simulink model "obstaculo_senoidal"  (R2025a)
settings: Solver=ode45  StartTime=0.0  StopTime=18  RelTol=1e-3
values from neighbouring files (symbols this model uses):
  a2 = entre_eixos - a_Ax    (= 0.114356)    [parametros_suspensao_completo_pibit_final.m]
  a_Ax = 0.070    (= 0.07)    [parametros_suspensao_completo_pibit_final.m]
  Hmax = 10/100    (= 0.1)    [parametros_suspensao_completo_pibit_final.m]
  Lqm = 3,7    [parametros_suspensao_completo_pibit_final.m]
  n_obs = 10    [parametros_suspensao_completo_pibit_final.m]
  Vv = 5    [parametros_suspensao_completo_pibit_final.m]
  Xobs = 10    [parametros_suspensao_completo_pibit_final.m]
libraries: simulink x4

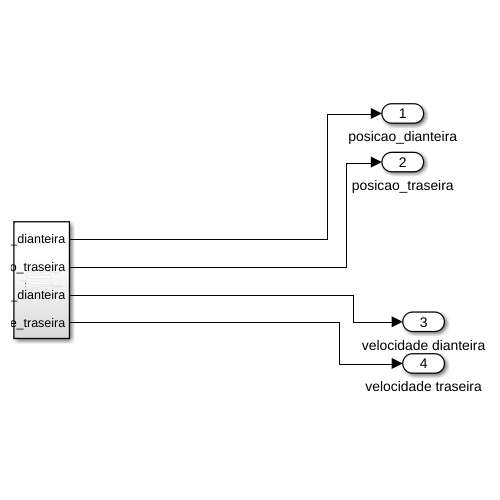
[thumbnail: Simulink's stored preview of the top-level diagram]
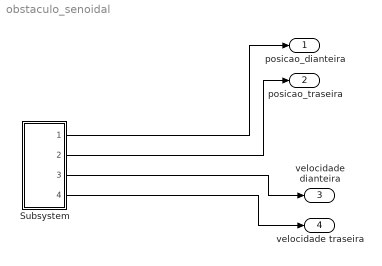
== system obstaculo_senoidal ==
  Subsystem : Subsystem
  posicao_dianteira : Outport
  posicao_traseira : Outport  Port=2
  velocidade dianteira : Outport  Port=3
  velocidade traseira : Outport  Port=4
  wires:
  Subsystem/1(posicao_dianteira) -> posicao_dianteira/1
  Subsystem/2(posicao_traseira) -> posicao_traseira/1
  Subsystem/3(velocidade_dianteira) -> velocidade dianteira/1
  Subsystem/4(velocidade_traseira) -> velocidade traseira/1

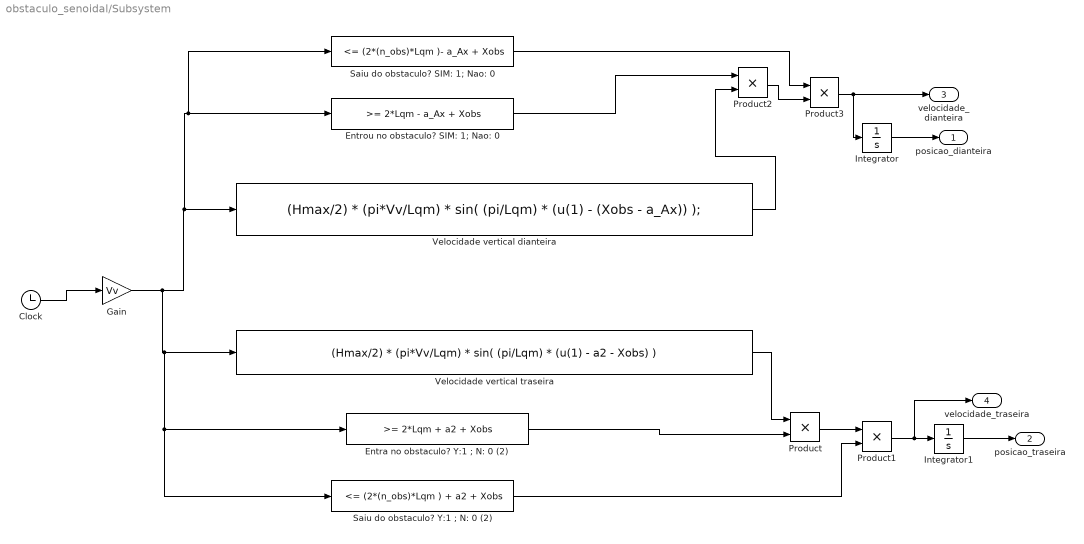
== system obstaculo_senoidal/Subsystem ==
  Clock : Clock
  Entra no obstaculo? Y:1 ; N: 0 (2) : simulink/Logic and Bit Operations/Compare To Constant  relop=>=  const=2*Lqm + a2 + Xobs  OutDataTypeStr=boolean
  "Entrou no obstaculo? SIM: 1; Nao: 0 " : simulink/Logic and Bit Operations/Compare To Constant  relop=>=  const=2*Lqm - a_Ax + Xobs  OutDataTypeStr=boolean
  Gain : Gain  Gain=Vv
  Integrator : Integrator
  Integrator1 : Integrator
  Product{,1..3} (4 alike) : Product
  "Saiu do obstaculo? SIM: 1; Nao: 0 " : simulink/Logic and Bit Operations/Compare To Constant  relop=<=  const=(2*(n_obs)*Lqm )- a_Ax + Xobs  OutDataTypeStr=boolean
  Saiu do obstaculo? Y:1 ; N: 0 (2) : simulink/Logic and Bit Operations/Compare To Constant  relop=<=  const=(2*(n_obs)*Lqm ) + a2 + Xobs  OutDataTypeStr=boolean
  Velocidade vertical dianteira : Fcn  Expr=(Hmax/2) * (pi*Vv/Lqm) * sin( (pi/Lqm) * (u(1) - (Xobs - a_Ax)) );
  Velocidade vertical traseira : Fcn  Expr=(Hmax/2) * (pi*Vv/Lqm) * sin( (pi/Lqm) * (u(1) - a2 - Xobs) )
  posicao_dianteira : Outport
  posicao_traseira : Outport  Port=2
  velocidade_dianteira : Outport  Port=3
  velocidade_traseira : Outport  Port=4
  wires:
  Gain/1 -> Saiu do obstaculo? Y:1 ; N: 0 (2)/1, Entra no obstaculo? Y:1 ; N: 0 (2)/1, Velocidade vertical traseira/1, "Saiu do obstaculo? SIM: 1; Nao: 0 "/1, "Entrou no obstaculo? SIM: 1; Nao: 0 "/1, Velocidade vertical dianteira/1
  Entra no obstaculo? Y:1 ; N: 0 (2)/1 -> Product/2
  "Saiu do obstaculo? SIM: 1; Nao: 0 "/1 -> Product3/1
  Saiu do obstaculo? Y:1 ; N: 0 (2)/1 -> Product1/2
  Product2/1 -> Product3/2
  Product3/1 -> velocidade_dianteira/1, Integrator/1
  Integrator/1 -> posicao_dianteira/1
  Product/1 -> Product1/1
  Velocidade vertical traseira/1 -> Product/1
  Product1/1 -> velocidade_traseira/1, Integrator1/1
  "Entrou no obstaculo? SIM: 1; Nao: 0 "/1 -> Product2/1
  Integrator1/1 -> posicao_traseira/1
  Velocidade vertical dianteira/1 -> Product2/2
  Clock/1 -> Gain/1
